simulink model "TorqueVect"  (R2022b)
settings: Solver=ode45  StartTime=0.0  StopTime=inf  RelTol=1e-3  EnableMultiTasking=on
undefined symbols (not defined in the file or in its folder): TC_Decr_Gas, TC_Derivative, TC_Incr_Gas, TC_On, TC_Relay_Off, TC_Relay_On, TV_On, TV_Override
libraries: CarMaker4SL x32, simulink x4, simulink_extras x4
(part 3 of 6)

== system TorqueVect/CarMaker/IPG Vehicle/CarAndTrailer/Forces/Suspension Forces/CreateBus FrcSystemCtrlOutOpt ==
  note: <Your model here>
  In : Inport
  Bus Creator9 : BusCreator  Inputs=64
  Demux : Demux  Outputs=64
  Out : Outport
  wires:
  In/1 -> Demux/1
  Bus Creator9/1 -> Out/1
  Demux/64 -> Bus Creator9/64  "CtrlOutOpt63"
  Demux/1 -> Bus Creator9/1  "CtrlOutOpt0"
  Demux/2 -> Bus Creator9/2  "CtrlOutOpt1"
  Demux/3 -> Bus Creator9/3  "CtrlOutOpt2"
  Demux/4 -> Bus Creator9/4  "CtrlOutOpt3"
  Demux/5 -> Bus Creator9/5  "CtrlOutOpt4"
  Demux/6 -> Bus Creator9/6  "CtrlOutOpt5"
  Demux/7 -> Bus Creator9/7  "CtrlOutOpt6"
  Demux/8 -> Bus Creator9/8  "CtrlOutOpt7"
  Demux/9 -> Bus Creator9/9  "CtrlOutOpt8"
  Demux/10 -> Bus Creator9/10  "CtrlOutOpt9"
  Demux/11 -> Bus Creator9/11  "CtrlOutOpt10"
  Demux/12 -> Bus Creator9/12  "CtrlOutOpt11"
  Demux/13 -> Bus Creator9/13  "CtrlOutOpt12"
  Demux/14 -> Bus Creator9/14  "CtrlOutOpt13"
  Demux/15 -> Bus Creator9/15  "CtrlOutOpt14"
  Demux/16 -> Bus Creator9/16  "CtrlOutOpt15"
  Demux/17 -> Bus Creator9/17  "CtrlOutOpt16"
  Demux/18 -> Bus Creator9/18  "CtrlOutOpt17"
  Demux/19 -> Bus Creator9/19  "CtrlOutOpt18"
  Demux/20 -> Bus Creator9/20  "CtrlOutOpt19"
  Demux/21 -> Bus Creator9/21  "CtrlOutOpt20"
  Demux/22 -> Bus Creator9/22  "CtrlOutOpt21"
  Demux/23 -> Bus Creator9/23  "CtrlOutOpt22"
  Demux/24 -> Bus Creator9/24  "CtrlOutOpt23"
  Demux/25 -> Bus Creator9/25  "CtrlOutOpt24"
  Demux/26 -> Bus Creator9/26  "CtrlOutOpt25"
  Demux/27 -> Bus Creator9/27  "CtrlOutOpt26"
  Demux/28 -> Bus Creator9/28  "CtrlOutOpt27"
  Demux/29 -> Bus Creator9/29  "CtrlOutOpt28"
  Demux/30 -> Bus Creator9/30  "CtrlOutOpt29"
  Demux/31 -> Bus Creator9/31  "CtrlOutOpt30"
  Demux/32 -> Bus Creator9/32  "CtrlOutOpt31"
  Demux/33 -> Bus Creator9/33  "CtrlOutOpt32"
  Demux/34 -> Bus Creator9/34  "CtrlOutOpt33"
  Demux/35 -> Bus Creator9/35  "CtrlOutOpt34"
  Demux/36 -> Bus Creator9/36  "CtrlOutOpt35"
  Demux/37 -> Bus Creator9/37  "CtrlOutOpt36"
  Demux/38 -> Bus Creator9/38  "CtrlOutOpt37"
  Demux/39 -> Bus Creator9/39  "CtrlOutOpt38"
  Demux/40 -> Bus Creator9/40  "CtrlOutOpt39"
  Demux/41 -> Bus Creator9/41  "CtrlOutOpt40"
  Demux/42 -> Bus Creator9/42  "CtrlOutOpt41"
  Demux/43 -> Bus Creator9/43  "CtrlOutOpt42"
  Demux/44 -> Bus Creator9/44  "CtrlOutOpt43"
  Demux/45 -> Bus Creator9/45  "CtrlOutOpt44"
  Demux/46 -> Bus Creator9/46  "CtrlOutOpt45"
  Demux/47 -> Bus Creator9/47  "CtrlOutOpt46"
  Demux/48 -> Bus Creator9/48  "CtrlOutOpt47"
  Demux/49 -> Bus Creator9/49  "CtrlOutOpt48"
  Demux/50 -> Bus Creator9/50  "CtrlOutOpt49"
  Demux/51 -> Bus Creator9/51  "CtrlOutOpt50"
  Demux/52 -> Bus Creator9/52  "CtrlOutOpt51"
  Demux/53 -> Bus Creator9/53  "CtrlOutOpt52"
  Demux/54 -> Bus Creator9/54  "CtrlOutOpt53"
  Demux/55 -> Bus Creator9/55  "CtrlOutOpt54"
  Demux/56 -> Bus Creator9/56  "CtrlOutOpt55"
  Demux/57 -> Bus Creator9/57  "CtrlOutOpt56"
  Demux/58 -> Bus Creator9/58  "CtrlOutOpt57"
  Demux/59 -> Bus Creator9/59  "CtrlOutOpt58"
  Demux/60 -> Bus Creator9/60  "CtrlOutOpt59"
  Demux/61 -> Bus Creator9/61  "CtrlOutOpt60"
  Demux/62 -> Bus Creator9/62  "CtrlOutOpt61"
  Demux/63 -> Bus Creator9/63  "CtrlOutOpt62"

== system TorqueVect/CarMaker/IPG Vehicle/CarAndTrailer/Forces/Suspension Forces/CreateBus SpringCtrlOutOpt ==
  note: <Your model here>
  In : Inport
  Bus Creator{,1..3,9} (5 alike) : BusCreator  Inputs=4
  Demux{,2..5} (5 alike) : Demux
  Out : Outport
  wires:
  Bus Creator/1 -> Bus Creator9/1
  Demux/4 -> Demux5/1  "RR"
  Bus Creator2/1 -> Bus Creator9/3
  Demux5/1 -> Bus Creator3/1  "RR CtrlOutOpt0"
  Bus Creator3/1 -> Bus Creator9/4
  Demux2/4 -> Bus Creator/4  "FL CtrlOutOpt3"
  Demux5/3 -> Bus Creator3/3  "RR CtrlOutOpt2"
  Demux4/3 -> Bus Creator2/3  "RL CtrlOutOpt2"
  Bus Creator1/1 -> Bus Creator9/2
  Demux4/2 -> Bus Creator2/2  "RL CtrlOutOpt1"
  Demux2/2 -> Bus Creator/2  "FL CtrlOutOpt1"
  Demux/2 -> Demux3/1  "FR"
  Demux3/4 -> Bus Creator1/4  "FR CtrlOutOpt3"
  Demux3/1 -> Bus Creator1/1  "FR CtrlOutOpt0"
  Demux4/4 -> Bus Creator2/4  "RL CtrlOutOpt3"
  Demux2/3 -> Bus Creator/3  "FL CtrlOutOpt2"
  Demux3/2 -> Bus Creator1/2  "FR CtrlOutOpt1"
  Demux2/1 -> Bus Creator/1  "FL CtrlOutOpt0"
  Demux3/3 -> Bus Creator1/3  "FR CtrlOutOpt2"
  In/1 -> Demux/1
  Demux5/4 -> Bus Creator3/4  "RR CtrlOutOpt3"
  Demux/3 -> Demux4/1  "RL"
  Bus Creator9/1 -> Out/1
  Demux5/2 -> Bus Creator3/2  "RR CtrlOutOpt1"
  Demux4/1 -> Bus Creator2/1  "RL CtrlOutOpt0"
  Demux/1 -> Demux2/1  "FL"

== system TorqueVect/CarMaker/IPG Vehicle/CarAndTrailer/Forces/Suspension Forces/CreateBus StabiCtrlOutOpt ==
  note: <Your model here>
  In : Inport
  Bus Creator{,1..3,9} (5 alike) : BusCreator  Inputs=4
  Demux{,2..5} (5 alike) : Demux
  Out : Outport
  wires:
  Bus Creator/1 -> Bus Creator9/1
  Demux/4 -> Demux5/1  "RR"
  Bus Creator2/1 -> Bus Creator9/3
  Demux5/1 -> Bus Creator3/1  "RR CtrlOutOpt0"
  Bus Creator3/1 -> Bus Creator9/4
  Demux2/4 -> Bus Creator/4  "FL CtrlOutOpt3"
  Demux5/3 -> Bus Creator3/3  "RR CtrlOutOpt2"
  Demux4/3 -> Bus Creator2/3  "RL CtrlOutOpt2"
  Bus Creator1/1 -> Bus Creator9/2
  Demux4/2 -> Bus Creator2/2  "RL CtrlOutOpt1"
  Demux2/2 -> Bus Creator/2  "FL CtrlOutOpt1"
  Demux/2 -> Demux3/1  "FR"
  Demux3/4 -> Bus Creator1/4  "FR CtrlOutOpt3"
  Demux3/1 -> Bus Creator1/1  "FR CtrlOutOpt0"
  Demux4/4 -> Bus Creator2/4  "RL CtrlOutOpt3"
  Demux2/3 -> Bus Creator/3  "FL CtrlOutOpt2"
  Demux3/2 -> Bus Creator1/2  "FR CtrlOutOpt1"
  Demux2/1 -> Bus Creator/1  "FL CtrlOutOpt0"
  Demux3/3 -> Bus Creator1/3  "FR CtrlOutOpt2"
  In/1 -> Demux/1
  Demux5/4 -> Bus Creator3/4  "RR CtrlOutOpt3"
  Demux/3 -> Demux4/1  "RL"
  Bus Creator9/1 -> Out/1
  Demux5/2 -> Bus Creator3/2  "RR CtrlOutOpt1"
  Demux4/1 -> Bus Creator2/1  "RL CtrlOutOpt0"
  Demux/1 -> Demux2/1  "FL"

== system TorqueVect/CarMaker/IPG Vehicle/CarAndTrailer/Forces/Suspension Forces/CreateBus Suspension Forces ==
  note: <Your model here>
  In : Inport
  Bus Creator10 : BusCreator  Inputs=4
  Bus Creator{4..7} (4 alike) : BusCreator  Inputs=6
  Demux1 : Demux
  Demux{6..9} (4 alike) : Demux  Outputs=6
  Out : Outport
  wires:
  Demux9/5 -> Bus Creator7/5  "RR ParasiticStiffForce"
  Demux9/4 -> Bus Creator7/4  "RR BufferForce"
  Demux6/5 -> Bus Creator4/5  "FL ParasiticStiffForce"
  Demux6/6 -> Bus Creator4/6  "FL ParasiticFricForce"
  Demux1/1 -> Demux6/1  "FL"
  Demux9/1 -> Bus Creator7/1  "RR SpringForce"
  Demux9/6 -> Bus Creator7/6  "RR ParasiticFricForce"
  Demux6/4 -> Bus Creator4/4  "FL BufferForce"
  Demux8/3 -> Bus Creator6/3  "RL StabiForce"
  Demux9/2 -> Bus Creator7/2  "RR DamperForce"
  Demux8/5 -> Bus Creator6/5  "RL ParasiticStiffForce"
  Bus Creator5/1 -> Bus Creator10/2
  Bus Creator6/1 -> Bus Creator10/3
  Bus Creator4/1 -> Bus Creator10/1
  Demux8/4 -> Bus Creator6/4  "RL BufferForce"
  Demux7/1 -> Bus Creator5/1  "FR SpringForce"
  Demux8/6 -> Bus Creator6/6  "RL ParasiticFricForce"
  Demux8/2 -> Bus Creator6/2  "RL DamperForce"
  Demux1/2 -> Demux7/1  "FR"
  Demux6/2 -> Bus Creator4/2  "FL DamperForce"
  Demux1/4 -> Demux9/1  "RR"
  Demux6/1 -> Bus Creator4/1  "FL SpringForce"
  Demux8/1 -> Bus Creator6/1  "RL SpringForce"
  Demux7/3 -> Bus Creator5/3  "FR StabiForce"
  In/1 -> Demux1/1
  Demux7/6 -> Bus Creator5/6  "FR ParasiticFricForce"
  Demux6/3 -> Bus Creator4/3  "FL StabiForce"
  Demux7/2 -> Bus Creator5/2  "FR DamperForce"
  Bus Creator10/1 -> Out/1
  Demux7/5 -> Bus Creator5/5  "FR ParasiticStiffForce"
  Demux7/4 -> Bus Creator5/4  "FR BufferForce"
  Demux9/3 -> Bus Creator7/3  "RR StabiForce"
  Demux1/3 -> Demux8/1  "RL"
  Bus Creator7/1 -> Bus Creator10/4

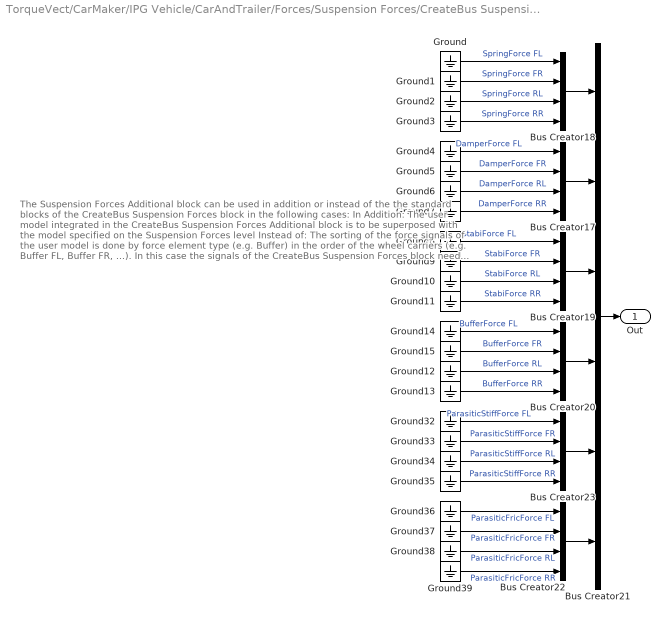
== system TorqueVect/CarMaker/IPG Vehicle/CarAndTrailer/Forces/Suspension Forces/CreateBus Suspension Forces Additional ==
  note: The Suspension Forces Additional block can be used in addition or instead of the
      | the standard blocks of the CreateBus Suspension Forces block in the following cases:
      |
      | In Addition: The user model integrated in the CreateBus Suspension Forces Additional block is to be superposed with the model specified on the Suspension Forces level
      | Instead of: The sorting of the force signals of the user model is done by force element type (e.g. Buffer) in the order of the wheel carriers (e.g. Buffer FL, Buffer FR, ...). In this case the signals of the CreateBus Suspension Forces block need to be disabled e.g. by manually connecting them to ground signals.
      |
      | ATTENTION : The forces given in the CreateBus Suspension Forces Additional block are internally added to the forces of the Suspension Forces block. If this is not desired, make sure to include a force model only in one of the two levels.
  Bus Creator{17..20,22..23} (6 alike) : BusCreator  Inputs=4
  Bus Creator21 : BusCreator  Inputs=6
  Ground{,1..15,32..39} (24 alike) : Ground
  Out : Outport
  wires:
  Ground1/1 -> Bus Creator18/2  "SpringForce FR"
  Ground9/1 -> Bus Creator19/2  "StabiForce FR"
  Ground8/1 -> Bus Creator19/1  "StabiForce FL"
  Bus Creator22/1 -> Bus Creator21/6
  Bus Creator21/1 -> Out/1
  Ground/1 -> Bus Creator18/1  "SpringForce FL"
  Ground36/1 -> Bus Creator22/1  "ParasiticFricForce FL"
  Ground2/1 -> Bus Creator18/3  "SpringForce RL"
  Ground5/1 -> Bus Creator17/2  "DamperForce FR"
  Ground15/1 -> Bus Creator20/2  "BufferForce FR"
  Ground35/1 -> Bus Creator23/4  "ParasiticStiffForce RR"
  Bus Creator20/1 -> Bus Creator21/4
  Bus Creator17/1 -> Bus Creator21/2
  Ground37/1 -> Bus Creator22/2  "ParasiticFricForce FR"
  Ground4/1 -> Bus Creator17/1  "DamperForce FL"
  Ground33/1 -> Bus Creator23/2  "ParasiticStiffForce FR"
  Bus Creator23/1 -> Bus Creator21/5
  Ground11/1 -> Bus Creator19/4  "StabiForce RR"
  Ground10/1 -> Bus Creator19/3  "StabiForce RL"
  Ground6/1 -> Bus Creator17/3  "DamperForce RL"
  Bus Creator19/1 -> Bus Creator21/3
  Ground7/1 -> Bus Creator17/4  "DamperForce RR"
  Bus Creator18/1 -> Bus Creator21/1
  Ground34/1 -> Bus Creator23/3  "ParasiticStiffForce RL"
  Ground3/1 -> Bus Creator18/4  "SpringForce RR"
  Ground12/1 -> Bus Creator20/3  "BufferForce RL"
  Ground38/1 -> Bus Creator22/3  "ParasiticFricForce RL"
  Ground14/1 -> Bus Creator20/1  "BufferForce FL"
  Ground39/1 -> Bus Creator22/4  "ParasiticFricForce RR"
  Ground32/1 -> Bus Creator23/1  "ParasiticStiffForce FL"
  Ground13/1 -> Bus Creator20/4  "BufferForce RR"

== system TorqueVect/CarMaker/IPG Vehicle/CarAndTrailer/Forces/Suspension Forces/CreateBus Suspension Forces CtrlOut ==
  note: <Your model here>
  In : Inport
  Bus Creator{,1..3,9} (5 alike) : BusCreator  Inputs=4
  Demux{,2..5} (5 alike) : Demux
  Out : Outport
  wires:
  Bus Creator3/1 -> Bus Creator9/4
  Demux2/4 -> Bus Creator/4  "FL BufferCtrlOut"
  Demux/4 -> Demux5/1  "RR"
  Bus Creator2/1 -> Bus Creator9/3
  Demux3/1 -> Bus Creator1/1  "FR SpringCtrlOut"
  Bus Creator/1 -> Bus Creator9/1
  Demux5/1 -> Bus Creator3/1  "RR SpringCtrlOut"
  Demux5/2 -> Bus Creator3/2  "RR DamperCtrlOut"
  Demux4/2 -> Bus Creator2/2  "RL DamperCtrlOut"
  Demux4/3 -> Bus Creator2/3  "RL StabiCtrlOut"
  Demux2/2 -> Bus Creator/2  "FL DamperCtrlOut"
  Demux/3 -> Demux4/1  "RL"
  Demux5/4 -> Bus Creator3/4  "RR BufferCtrlOut"
  In/1 -> Demux/1
  Demux2/1 -> Bus Creator/1  "FL SpringCtrlOut"
  Demux3/3 -> Bus Creator1/3  "FR StabiCtrlOut"
  Demux3/2 -> Bus Creator1/2  "FR DamperCtrlOut"
  Demux4/1 -> Bus Creator2/1  "RL SpringCtrlOut"
  Demux4/4 -> Bus Creator2/4  "RL BufferCtrlOut"
  Demux2/3 -> Bus Creator/3  "FL StabiCtrlOut"
  Bus Creator1/1 -> Bus Creator9/2
  Bus Creator9/1 -> Out/1
  Demux/1 -> Demux2/1  "FL"
  Demux/2 -> Demux3/1  "FR"
  Demux5/3 -> Bus Creator3/3  "RR StabiCtrlOut"
  Demux3/4 -> Bus Creator1/4  "FR BufferCtrlOut"

== system TorqueVect/CarMaker/IPG Vehicle/CarAndTrailer/Forces/Suspension Forces/Damper CreateBus CtrlOutOpt ==
  note: <Your model here>
  In : Inport
  Bus Creator{,1..3,9} (5 alike) : BusCreator  Inputs=4
  Demux{,2..5} (5 alike) : Demux
  Out : Outport
  wires:
  Bus Creator/1 -> Bus Creator9/1
  Demux/4 -> Demux5/1  "RR"
  Bus Creator2/1 -> Bus Creator9/3
  Demux5/1 -> Bus Creator3/1  "RR CtrlOutOpt0"
  Bus Creator3/1 -> Bus Creator9/4
  Demux2/4 -> Bus Creator/4  "FL CtrlOutOpt3"
  Demux5/3 -> Bus Creator3/3  "RR CtrlOutOpt2"
  Demux4/3 -> Bus Creator2/3  "RL CtrlOutOpt2"
  Bus Creator1/1 -> Bus Creator9/2
  Demux4/2 -> Bus Creator2/2  "RL CtrlOutOpt1"
  Demux2/2 -> Bus Creator/2  "FL CtrlOutOpt1"
  Demux/2 -> Demux3/1  "FR"
  Demux3/4 -> Bus Creator1/4  "FR CtrlOutOpt3"
  Demux3/1 -> Bus Creator1/1  "FR CtrlOutOpt0"
  Demux4/4 -> Bus Creator2/4  "RL CtrlOutOpt3"
  Demux2/3 -> Bus Creator/3  "FL CtrlOutOpt2"
  Demux3/2 -> Bus Creator1/2  "FR CtrlOutOpt1"
  Demux2/1 -> Bus Creator/1  "FL CtrlOutOpt0"
  Demux3/3 -> Bus Creator1/3  "FR CtrlOutOpt2"
  In/1 -> Demux/1
  Demux5/4 -> Bus Creator3/4  "RR CtrlOutOpt3"
  Demux/3 -> Demux4/1  "RL"
  Bus Creator9/1 -> Out/1
  Demux5/2 -> Bus Creator3/2  "RR CtrlOutOpt1"
  Demux4/1 -> Bus Creator2/1  "RL CtrlOutOpt0"
  Demux/1 -> Demux2/1  "FL"

== system TorqueVect/CarMaker/IPG Vehicle/CarAndTrailer/Forces/Suspension Forces/FrcSystem CreateBus CtrlOutOpt ==
  note: <Your model here>
  In : Inport
  Bus Creator9 : BusCreator  Inputs=64
  Demux : Demux  Outputs=64
  Out : Outport
  wires:
  In/1 -> Demux/1
  Bus Creator9/1 -> Out/1
  Demux/64 -> Bus Creator9/64  "CtrlOutOpt63"
  Demux/1 -> Bus Creator9/1  "CtrlOutOpt0"
  Demux/2 -> Bus Creator9/2  "CtrlOutOpt1"
  Demux/3 -> Bus Creator9/3  "CtrlOutOpt2"
  Demux/4 -> Bus Creator9/4  "CtrlOutOpt3"
  Demux/5 -> Bus Creator9/5  "CtrlOutOpt4"
  Demux/6 -> Bus Creator9/6  "CtrlOutOpt5"
  Demux/7 -> Bus Creator9/7  "CtrlOutOpt6"
  Demux/8 -> Bus Creator9/8  "CtrlOutOpt7"
  Demux/9 -> Bus Creator9/9  "CtrlOutOpt8"
  Demux/10 -> Bus Creator9/10  "CtrlOutOpt9"
  Demux/11 -> Bus Creator9/11  "CtrlOutOpt10"
  Demux/12 -> Bus Creator9/12  "CtrlOutOpt11"
  Demux/13 -> Bus Creator9/13  "CtrlOutOpt12"
  Demux/14 -> Bus Creator9/14  "CtrlOutOpt13"
  Demux/15 -> Bus Creator9/15  "CtrlOutOpt14"
  Demux/16 -> Bus Creator9/16  "CtrlOutOpt15"
  Demux/17 -> Bus Creator9/17  "CtrlOutOpt16"
  Demux/18 -> Bus Creator9/18  "CtrlOutOpt17"
  Demux/19 -> Bus Creator9/19  "CtrlOutOpt18"
  Demux/20 -> Bus Creator9/20  "CtrlOutOpt19"
  Demux/21 -> Bus Creator9/21  "CtrlOutOpt20"
  Demux/22 -> Bus Creator9/22  "CtrlOutOpt21"
  Demux/23 -> Bus Creator9/23  "CtrlOutOpt22"
  Demux/24 -> Bus Creator9/24  "CtrlOutOpt23"
  Demux/25 -> Bus Creator9/25  "CtrlOutOpt24"
  Demux/26 -> Bus Creator9/26  "CtrlOutOpt25"
  Demux/27 -> Bus Creator9/27  "CtrlOutOpt26"
  Demux/28 -> Bus Creator9/28  "CtrlOutOpt27"
  Demux/29 -> Bus Creator9/29  "CtrlOutOpt28"
  Demux/30 -> Bus Creator9/30  "CtrlOutOpt29"
  Demux/31 -> Bus Creator9/31  "CtrlOutOpt30"
  Demux/32 -> Bus Creator9/32  "CtrlOutOpt31"
  Demux/33 -> Bus Creator9/33  "CtrlOutOpt32"
  Demux/34 -> Bus Creator9/34  "CtrlOutOpt33"
  Demux/35 -> Bus Creator9/35  "CtrlOutOpt34"
  Demux/36 -> Bus Creator9/36  "CtrlOutOpt35"
  Demux/37 -> Bus Creator9/37  "CtrlOutOpt36"
  Demux/38 -> Bus Creator9/38  "CtrlOutOpt37"
  Demux/39 -> Bus Creator9/39  "CtrlOutOpt38"
  Demux/40 -> Bus Creator9/40  "CtrlOutOpt39"
  Demux/41 -> Bus Creator9/41  "CtrlOutOpt40"
  Demux/42 -> Bus Creator9/42  "CtrlOutOpt41"
  Demux/43 -> Bus Creator9/43  "CtrlOutOpt42"
  Demux/44 -> Bus Creator9/44  "CtrlOutOpt43"
  Demux/45 -> Bus Creator9/45  "CtrlOutOpt44"
  Demux/46 -> Bus Creator9/46  "CtrlOutOpt45"
  Demux/47 -> Bus Creator9/47  "CtrlOutOpt46"
  Demux/48 -> Bus Creator9/48  "CtrlOutOpt47"
  Demux/49 -> Bus Creator9/49  "CtrlOutOpt48"
  Demux/50 -> Bus Creator9/50  "CtrlOutOpt49"
  Demux/51 -> Bus Creator9/51  "CtrlOutOpt50"
  Demux/52 -> Bus Creator9/52  "CtrlOutOpt51"
  Demux/53 -> Bus Creator9/53  "CtrlOutOpt52"
  Demux/54 -> Bus Creator9/54  "CtrlOutOpt53"
  Demux/55 -> Bus Creator9/55  "CtrlOutOpt54"
  Demux/56 -> Bus Creator9/56  "CtrlOutOpt55"
  Demux/57 -> Bus Creator9/57  "CtrlOutOpt56"
  Demux/58 -> Bus Creator9/58  "CtrlOutOpt57"
  Demux/59 -> Bus Creator9/59  "CtrlOutOpt58"
  Demux/60 -> Bus Creator9/60  "CtrlOutOpt59"
  Demux/61 -> Bus Creator9/61  "CtrlOutOpt60"
  Demux/62 -> Bus Creator9/62  "CtrlOutOpt61"
  Demux/63 -> Bus Creator9/63  "CtrlOutOpt62"

== system TorqueVect/CarMaker/IPG Vehicle/CarAndTrailer/Forces/Suspension Forces/Spring CreateBus CtrlOutOpt ==
  note: <Your model here>
  In : Inport
  Bus Creator{,1..3,9} (5 alike) : BusCreator  Inputs=4
  Demux{,2..5} (5 alike) : Demux
  Out : Outport
  wires:
  Bus Creator/1 -> Bus Creator9/1
  Demux/4 -> Demux5/1  "RR"
  Bus Creator2/1 -> Bus Creator9/3
  Demux5/1 -> Bus Creator3/1  "RR CtrlOutOpt0"
  Bus Creator3/1 -> Bus Creator9/4
  Demux2/4 -> Bus Creator/4  "FL CtrlOutOpt3"
  Demux5/3 -> Bus Creator3/3  "RR CtrlOutOpt2"
  Demux4/3 -> Bus Creator2/3  "RL CtrlOutOpt2"
  Bus Creator1/1 -> Bus Creator9/2
  Demux4/2 -> Bus Creator2/2  "RL CtrlOutOpt1"
  Demux2/2 -> Bus Creator/2  "FL CtrlOutOpt1"
  Demux/2 -> Demux3/1  "FR"
  Demux3/4 -> Bus Creator1/4  "FR CtrlOutOpt3"
  Demux3/1 -> Bus Creator1/1  "FR CtrlOutOpt0"
  Demux4/4 -> Bus Creator2/4  "RL CtrlOutOpt3"
  Demux2/3 -> Bus Creator/3  "FL CtrlOutOpt2"
  Demux3/2 -> Bus Creator1/2  "FR CtrlOutOpt1"
  Demux2/1 -> Bus Creator/1  "FL CtrlOutOpt0"
  Demux3/3 -> Bus Creator1/3  "FR CtrlOutOpt2"
  In/1 -> Demux/1
  Demux5/4 -> Bus Creator3/4  "RR CtrlOutOpt3"
  Demux/3 -> Demux4/1  "RL"
  Bus Creator9/1 -> Out/1
  Demux5/2 -> Bus Creator3/2  "RR CtrlOutOpt1"
  Demux4/1 -> Bus Creator2/1  "RL CtrlOutOpt0"
  Demux/1 -> Demux2/1  "FL"

== system TorqueVect/CarMaker/IPG Vehicle/CarAndTrailer/Forces/Suspension Forces/Stabi CreateBus CtrlOutOpt ==
  note: <Your model here>
  In : Inport
  Bus Creator{,1..3,9} (5 alike) : BusCreator  Inputs=4
  Demux{,2..5} (5 alike) : Demux
  Out : Outport
  wires:
  Bus Creator/1 -> Bus Creator9/1
  Demux/4 -> Demux5/1  "RR"
  Bus Creator2/1 -> Bus Creator9/3
  Demux5/1 -> Bus Creator3/1  "RR CtrlOutOpt0"
  Bus Creator3/1 -> Bus Creator9/4
  Demux2/4 -> Bus Creator/4  "FL CtrlOutOpt3"
  Demux5/3 -> Bus Creator3/3  "RR CtrlOutOpt2"
  Demux4/3 -> Bus Creator2/3  "RL CtrlOutOpt2"
  Bus Creator1/1 -> Bus Creator9/2
  Demux4/2 -> Bus Creator2/2  "RL CtrlOutOpt1"
  Demux2/2 -> Bus Creator/2  "FL CtrlOutOpt1"
  Demux/2 -> Demux3/1  "FR"
  Demux3/4 -> Bus Creator1/4  "FR CtrlOutOpt3"
  Demux3/1 -> Bus Creator1/1  "FR CtrlOutOpt0"
  Demux4/4 -> Bus Creator2/4  "RL CtrlOutOpt3"
  Demux2/3 -> Bus Creator/3  "FL CtrlOutOpt2"
  Demux3/2 -> Bus Creator1/2  "FR CtrlOutOpt1"
  Demux2/1 -> Bus Creator/1  "FL CtrlOutOpt0"
  Demux3/3 -> Bus Creator1/3  "FR CtrlOutOpt2"
  In/1 -> Demux/1
  Demux5/4 -> Bus Creator3/4  "RR CtrlOutOpt3"
  Demux/3 -> Demux4/1  "RL"
  Bus Creator9/1 -> Out/1
  Demux5/2 -> Bus Creator3/2  "RR CtrlOutOpt1"
  Demux4/1 -> Bus Creator2/1  "RL CtrlOutOpt0"
  Demux/1 -> Demux2/1  "FL"

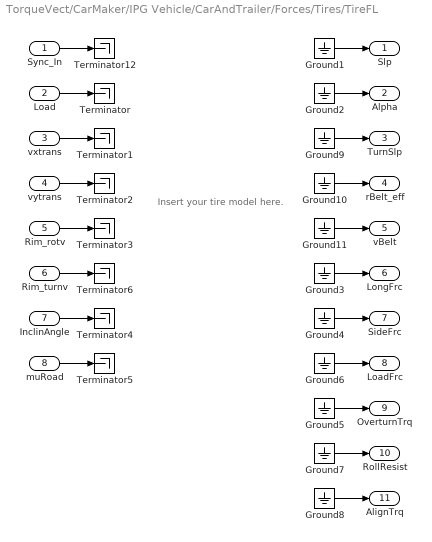
== system TorqueVect/CarMaker/IPG Vehicle/CarAndTrailer/Forces/Tires/TireFL ==
  note: Insert your tire model here.
  Sync_In : Inport
  Load : Inport  Port=2
  vxtrans : Inport  Port=3
  vytrans : Inport  Port=4
  Rim_rotv : Inport  Port=5
  Rim_turnv : Inport  Port=6
  InclinAngle : Inport  Port=7
  muRoad : Inport  Port=8
  Ground{1..11} (11 alike) : Ground
  Terminator{,1..6,12} (8 alike) : Terminator
  Slp : Outport  VectorParamsAs1DForOutWhenUnconnected=off
  Alpha : Outport  Port=2  VectorParamsAs1DForOutWhenUnconnected=off
  TurnSlp : Outport  Port=3  VectorParamsAs1DForOutWhenUnconnected=off
  rBelt_eff : Outport  Port=4  VectorParamsAs1DForOutWhenUnconnected=off
  vBelt : Outport  Port=5  VectorParamsAs1DForOutWhenUnconnected=off
  LongFrc : Outport  Port=6  VectorParamsAs1DForOutWhenUnconnected=off
  SideFrc : Outport  Port=7  VectorParamsAs1DForOutWhenUnconnected=off
  LoadFrc : Outport  Port=8  VectorParamsAs1DForOutWhenUnconnected=off
  OverturnTrq : Outport  Port=9  VectorParamsAs1DForOutWhenUnconnected=off
  RollResist : Outport  Port=10  VectorParamsAs1DForOutWhenUnconnected=off
  AlignTrq : Outport  Port=11  VectorParamsAs1DForOutWhenUnconnected=off
  wires:
  Ground11/1 -> vBelt/1
  Ground10/1 -> rBelt_eff/1
  Ground9/1 -> TurnSlp/1
  Rim_turnv/1 -> Terminator6/1
  Sync_In/1 -> Terminator12/1
  Ground2/1 -> Alpha/1
  Ground3/1 -> LongFrc/1
  Ground4/1 -> SideFrc/1
  Ground5/1 -> OverturnTrq/1
  vxtrans/1 -> Terminator1/1
  vytrans/1 -> Terminator2/1
  Rim_rotv/1 -> Terminator3/1
  InclinAngle/1 -> Terminator4/1
  muRoad/1 -> Terminator5/1
  Load/1 -> Terminator/1
  Ground1/1 -> Slp/1
  Ground6/1 -> LoadFrc/1
  Ground7/1 -> RollResist/1
  Ground8/1 -> AlignTrq/1

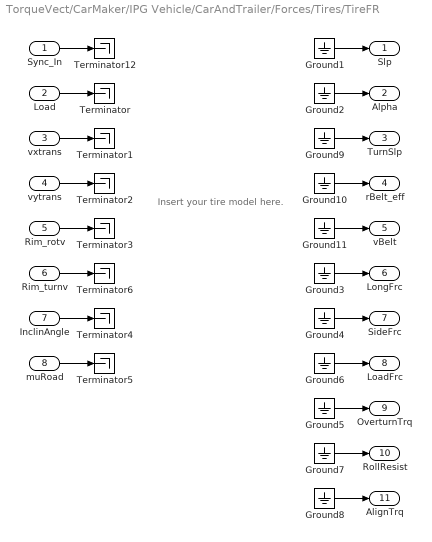
== system TorqueVect/CarMaker/IPG Vehicle/CarAndTrailer/Forces/Tires/TireFR ==
  note: Insert your tire model here.
  Sync_In : Inport
  Load : Inport  Port=2
  vxtrans : Inport  Port=3
  vytrans : Inport  Port=4
  Rim_rotv : Inport  Port=5
  Rim_turnv : Inport  Port=6
  InclinAngle : Inport  Port=7
  muRoad : Inport  Port=8
  Ground{1..11} (11 alike) : Ground
  Terminator{,1..6,12} (8 alike) : Terminator
  Slp : Outport  VectorParamsAs1DForOutWhenUnconnected=off
  Alpha : Outport  Port=2  VectorParamsAs1DForOutWhenUnconnected=off
  TurnSlp : Outport  Port=3  VectorParamsAs1DForOutWhenUnconnected=off
  rBelt_eff : Outport  Port=4  VectorParamsAs1DForOutWhenUnconnected=off
  vBelt : Outport  Port=5  VectorParamsAs1DForOutWhenUnconnected=off
  LongFrc : Outport  Port=6  VectorParamsAs1DForOutWhenUnconnected=off
  SideFrc : Outport  Port=7  VectorParamsAs1DForOutWhenUnconnected=off
  LoadFrc : Outport  Port=8  VectorParamsAs1DForOutWhenUnconnected=off
  OverturnTrq : Outport  Port=9  VectorParamsAs1DForOutWhenUnconnected=off
  RollResist : Outport  Port=10  VectorParamsAs1DForOutWhenUnconnected=off
  AlignTrq : Outport  Port=11  VectorParamsAs1DForOutWhenUnconnected=off
  wires:
  Ground11/1 -> vBelt/1
  Ground10/1 -> rBelt_eff/1
  Ground9/1 -> TurnSlp/1
  Rim_turnv/1 -> Terminator6/1
  Sync_In/1 -> Terminator12/1
  Ground2/1 -> Alpha/1
  Ground3/1 -> LongFrc/1
  Ground4/1 -> SideFrc/1
  Ground5/1 -> OverturnTrq/1
  vxtrans/1 -> Terminator1/1
  vytrans/1 -> Terminator2/1
  Rim_rotv/1 -> Terminator3/1
  InclinAngle/1 -> Terminator4/1
  muRoad/1 -> Terminator5/1
  Load/1 -> Terminator/1
  Ground1/1 -> Slp/1
  Ground6/1 -> LoadFrc/1
  Ground7/1 -> RollResist/1
  Ground8/1 -> AlignTrq/1

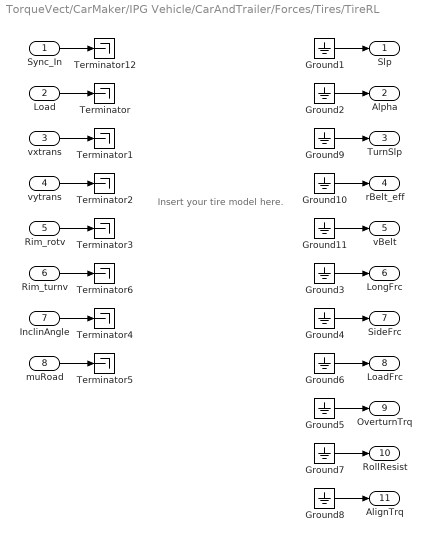
== system TorqueVect/CarMaker/IPG Vehicle/CarAndTrailer/Forces/Tires/TireRL ==
  note: Insert your tire model here.
  Sync_In : Inport
  Load : Inport  Port=2
  vxtrans : Inport  Port=3
  vytrans : Inport  Port=4
  Rim_rotv : Inport  Port=5
  Rim_turnv : Inport  Port=6
  InclinAngle : Inport  Port=7
  muRoad : Inport  Port=8
  Ground{1..11} (11 alike) : Ground
  Terminator{,1..6,12} (8 alike) : Terminator
  Slp : Outport  VectorParamsAs1DForOutWhenUnconnected=off
  Alpha : Outport  Port=2  VectorParamsAs1DForOutWhenUnconnected=off
  TurnSlp : Outport  Port=3  VectorParamsAs1DForOutWhenUnconnected=off
  rBelt_eff : Outport  Port=4  VectorParamsAs1DForOutWhenUnconnected=off
  vBelt : Outport  Port=5  VectorParamsAs1DForOutWhenUnconnected=off
  LongFrc : Outport  Port=6  VectorParamsAs1DForOutWhenUnconnected=off
  SideFrc : Outport  Port=7  VectorParamsAs1DForOutWhenUnconnected=off
  LoadFrc : Outport  Port=8  VectorParamsAs1DForOutWhenUnconnected=off
  OverturnTrq : Outport  Port=9  VectorParamsAs1DForOutWhenUnconnected=off
  RollResist : Outport  Port=10  VectorParamsAs1DForOutWhenUnconnected=off
  AlignTrq : Outport  Port=11  VectorParamsAs1DForOutWhenUnconnected=off
  wires:
  Ground11/1 -> vBelt/1
  Ground10/1 -> rBelt_eff/1
  Ground9/1 -> TurnSlp/1
  Rim_turnv/1 -> Terminator6/1
  Sync_In/1 -> Terminator12/1
  Ground2/1 -> Alpha/1
  Ground3/1 -> LongFrc/1
  Ground4/1 -> SideFrc/1
  Ground5/1 -> OverturnTrq/1
  vxtrans/1 -> Terminator1/1
  vytrans/1 -> Terminator2/1
  Rim_rotv/1 -> Terminator3/1
  InclinAngle/1 -> Terminator4/1
  muRoad/1 -> Terminator5/1
  Load/1 -> Terminator/1
  Ground1/1 -> Slp/1
  Ground6/1 -> LoadFrc/1
  Ground7/1 -> RollResist/1
  Ground8/1 -> AlignTrq/1

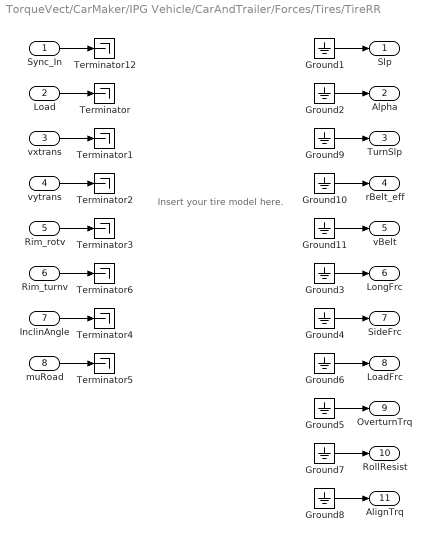
== system TorqueVect/CarMaker/IPG Vehicle/CarAndTrailer/Forces/Tires/TireRR ==
  note: Insert your tire model here.
  Sync_In : Inport
  Load : Inport  Port=2
  vxtrans : Inport  Port=3
  vytrans : Inport  Port=4
  Rim_rotv : Inport  Port=5
  Rim_turnv : Inport  Port=6
  InclinAngle : Inport  Port=7
  muRoad : Inport  Port=8
  Ground{1..11} (11 alike) : Ground
  Terminator{,1..6,12} (8 alike) : Terminator
  Slp : Outport  VectorParamsAs1DForOutWhenUnconnected=off
  Alpha : Outport  Port=2  VectorParamsAs1DForOutWhenUnconnected=off
  TurnSlp : Outport  Port=3  VectorParamsAs1DForOutWhenUnconnected=off
  rBelt_eff : Outport  Port=4  VectorParamsAs1DForOutWhenUnconnected=off
  vBelt : Outport  Port=5  VectorParamsAs1DForOutWhenUnconnected=off
  LongFrc : Outport  Port=6  VectorParamsAs1DForOutWhenUnconnected=off
  SideFrc : Outport  Port=7  VectorParamsAs1DForOutWhenUnconnected=off
  LoadFrc : Outport  Port=8  VectorParamsAs1DForOutWhenUnconnected=off
  OverturnTrq : Outport  Port=9  VectorParamsAs1DForOutWhenUnconnected=off
  RollResist : Outport  Port=10  VectorParamsAs1DForOutWhenUnconnected=off
  AlignTrq : Outport  Port=11  VectorParamsAs1DForOutWhenUnconnected=off
  wires:
  Ground11/1 -> vBelt/1
  Ground10/1 -> rBelt_eff/1
  Ground9/1 -> TurnSlp/1
  Rim_turnv/1 -> Terminator6/1
  Sync_In/1 -> Terminator12/1
  Ground2/1 -> Alpha/1
  Ground3/1 -> LongFrc/1
  Ground4/1 -> SideFrc/1
  Ground5/1 -> OverturnTrq/1
  vxtrans/1 -> Terminator1/1
  vytrans/1 -> Terminator2/1
  Rim_rotv/1 -> Terminator3/1
  InclinAngle/1 -> Terminator4/1
  muRoad/1 -> Terminator5/1
  Load/1 -> Terminator/1
  Ground1/1 -> Slp/1
  Ground6/1 -> LoadFrc/1
  Ground7/1 -> RollResist/1
  Ground8/1 -> AlignTrq/1

== system TorqueVect/CarMaker/IPG Vehicle/PowerTrain/PTControl Example/PTC ClutchOut/CreateBus PTC ClutchOut0 ==
  In : Inport
  BusCreator : BusCreator  Inputs=3
  Demux : Demux  Outputs=3
      settings: DisplayOption=none
  Out : Outport  VectorParamsAs1DForOutWhenUnconnected=off
  wires:
  Demux/3 -> BusCreator/3  "PTC ClutchOut0 Trq_out_trg"
  Demux/2 -> BusCreator/2  "PTC ClutchOut0 rotv_out_trg"
  Demux/1 -> BusCreator/1  "PTC ClutchOut0 Pos"
  BusCreator/1 -> Out/1
  In/1 -> Demux/1

== system TorqueVect/CarMaker/IPG Vehicle/PowerTrain/PTControl Example/PTC ClutchOut/CreateBus PTC ClutchOut1 ==
  In : Inport
  BusCreator : BusCreator  Inputs=3
  Demux : Demux  Outputs=3
      settings: DisplayOption=none
  Out : Outport  VectorParamsAs1DForOutWhenUnconnected=off
  wires:
  Demux/3 -> BusCreator/3  "PTC ClutchOut1 Trq_out_trg"
  Demux/2 -> BusCreator/2  "PTC ClutchOut1 rotv_out_trg"
  Demux/1 -> BusCreator/1  "PTC ClutchOut1 Pos"
  BusCreator/1 -> Out/1
  In/1 -> Demux/1

== system TorqueVect/CarMaker/IPG Vehicle/PowerTrain/PTControl Example/PTC ClutchOut/CreateBus PTC ClutchOut10 ==
  In : Inport
  BusCreator : BusCreator  Inputs=3
  Demux : Demux  Outputs=3
      settings: DisplayOption=none
  Out : Outport  VectorParamsAs1DForOutWhenUnconnected=off
  wires:
  Demux/3 -> BusCreator/3  "PTC ClutchOut10 Trq_out_trg"
  Demux/2 -> BusCreator/2  "PTC ClutchOut10 rotv_out_trg"
  Demux/1 -> BusCreator/1  "PTC ClutchOut10 Pos"
  BusCreator/1 -> Out/1
  In/1 -> Demux/1

== system TorqueVect/CarMaker/IPG Vehicle/PowerTrain/PTControl Example/PTC ClutchOut/CreateBus PTC ClutchOut11 ==
  In : Inport
  BusCreator : BusCreator  Inputs=3
  Demux : Demux  Outputs=3
      settings: DisplayOption=none
  Out : Outport  VectorParamsAs1DForOutWhenUnconnected=off
  wires:
  Demux/3 -> BusCreator/3  "PTC ClutchOut11 Trq_out_trg"
  Demux/2 -> BusCreator/2  "PTC ClutchOut11 rotv_out_trg"
  Demux/1 -> BusCreator/1  "PTC ClutchOut11 Pos"
  BusCreator/1 -> Out/1
  In/1 -> Demux/1

== system TorqueVect/CarMaker/IPG Vehicle/PowerTrain/PTControl Example/PTC ClutchOut/CreateBus PTC ClutchOut2 ==
  In : Inport
  BusCreator : BusCreator  Inputs=3
  Demux : Demux  Outputs=3
      settings: DisplayOption=none
  Out : Outport  VectorParamsAs1DForOutWhenUnconnected=off
  wires:
  Demux/3 -> BusCreator/3  "PTC ClutchOut2 Trq_out_trg"
  Demux/2 -> BusCreator/2  "PTC ClutchOut2 rotv_out_trg"
  Demux/1 -> BusCreator/1  "PTC ClutchOut2 Pos"
  BusCreator/1 -> Out/1
  In/1 -> Demux/1

== system TorqueVect/CarMaker/IPG Vehicle/PowerTrain/PTControl Example/PTC ClutchOut/CreateBus PTC ClutchOut3 ==
  In : Inport
  BusCreator : BusCreator  Inputs=3
  Demux : Demux  Outputs=3
      settings: DisplayOption=none
  Out : Outport  VectorParamsAs1DForOutWhenUnconnected=off
  wires:
  Demux/3 -> BusCreator/3  "PTC ClutchOut3 Trq_out_trg"
  Demux/2 -> BusCreator/2  "PTC ClutchOut3 rotv_out_trg"
  Demux/1 -> BusCreator/1  "PTC ClutchOut3 Pos"
  BusCreator/1 -> Out/1
  In/1 -> Demux/1

== system TorqueVect/CarMaker/IPG Vehicle/PowerTrain/PTControl Example/PTC ClutchOut/CreateBus PTC ClutchOut4 ==
  In : Inport
  BusCreator : BusCreator  Inputs=3
  Demux : Demux  Outputs=3
      settings: DisplayOption=none
  Out : Outport  VectorParamsAs1DForOutWhenUnconnected=off
  wires:
  Demux/3 -> BusCreator/3  "PTC ClutchOut4 Trq_out_trg"
  Demux/2 -> BusCreator/2  "PTC ClutchOut4 rotv_out_trg"
  Demux/1 -> BusCreator/1  "PTC ClutchOut4 Pos"
  BusCreator/1 -> Out/1
  In/1 -> Demux/1

== system TorqueVect/CarMaker/IPG Vehicle/PowerTrain/PTControl Example/PTC ClutchOut/CreateBus PTC ClutchOut5 ==
  In : Inport
  BusCreator : BusCreator  Inputs=3
  Demux : Demux  Outputs=3
      settings: DisplayOption=none
  Out : Outport  VectorParamsAs1DForOutWhenUnconnected=off
  wires:
  Demux/3 -> BusCreator/3  "PTC ClutchOut5 Trq_out_trg"
  Demux/2 -> BusCreator/2  "PTC ClutchOut5 rotv_out_trg"
  Demux/1 -> BusCreator/1  "PTC ClutchOut5 Pos"
  BusCreator/1 -> Out/1
  In/1 -> Demux/1

== system TorqueVect/CarMaker/IPG Vehicle/PowerTrain/PTControl Example/PTC ClutchOut/CreateBus PTC ClutchOut6 ==
  In : Inport
  BusCreator : BusCreator  Inputs=3
  Demux : Demux  Outputs=3
      settings: DisplayOption=none
  Out : Outport  VectorParamsAs1DForOutWhenUnconnected=off
  wires:
  Demux/3 -> BusCreator/3  "PTC ClutchOut6 Trq_out_trg"
  Demux/2 -> BusCreator/2  "PTC ClutchOut6 rotv_out_trg"
  Demux/1 -> BusCreator/1  "PTC ClutchOut6 Pos"
  BusCreator/1 -> Out/1
  In/1 -> Demux/1

== system TorqueVect/CarMaker/IPG Vehicle/PowerTrain/PTControl Example/PTC ClutchOut/CreateBus PTC ClutchOut7 ==
  In : Inport
  BusCreator : BusCreator  Inputs=3
  Demux : Demux  Outputs=3
      settings: DisplayOption=none
  Out : Outport  VectorParamsAs1DForOutWhenUnconnected=off
  wires:
  Demux/3 -> BusCreator/3  "PTC ClutchOut7 Trq_out_trg"
  Demux/2 -> BusCreator/2  "PTC ClutchOut7 rotv_out_trg"
  Demux/1 -> BusCreator/1  "PTC ClutchOut7 Pos"
  BusCreator/1 -> Out/1
  In/1 -> Demux/1

== system TorqueVect/CarMaker/IPG Vehicle/PowerTrain/PTControl Example/PTC ClutchOut/CreateBus PTC ClutchOut8 ==
  In : Inport
  BusCreator : BusCreator  Inputs=3
  Demux : Demux  Outputs=3
      settings: DisplayOption=none
  Out : Outport  VectorParamsAs1DForOutWhenUnconnected=off
  wires:
  Demux/3 -> BusCreator/3  "PTC ClutchOut8 Trq_out_trg"
  Demux/2 -> BusCreator/2  "PTC ClutchOut8 rotv_out_trg"
  Demux/1 -> BusCreator/1  "PTC ClutchOut8 Pos"
  BusCreator/1 -> Out/1
  In/1 -> Demux/1

== system TorqueVect/CarMaker/IPG Vehicle/PowerTrain/PTControl Example/PTC ClutchOut/CreateBus PTC ClutchOut9 ==
  In : Inport
  BusCreator : BusCreator  Inputs=3
  Demux : Demux  Outputs=3
      settings: DisplayOption=none
  Out : Outport  VectorParamsAs1DForOutWhenUnconnected=off
  wires:
  Demux/3 -> BusCreator/3  "PTC ClutchOut9 Trq_out_trg"
  Demux/2 -> BusCreator/2  "PTC ClutchOut9 rotv_out_trg"
  Demux/1 -> BusCreator/1  "PTC ClutchOut9 Pos"
  BusCreator/1 -> Out/1
  In/1 -> Demux/1

== system TorqueVect/CarMaker/IPG Vehicle/PowerTrain/PTControl Example/PTC GearBoxOut/CreateBus PTC GearboxOut0 ==
  In : Inport
  BusCreator : BusCreator  Inputs=12
  Demux : Demux  Outputs=12
      settings: DisplayOption=none
  Out : Outport  VectorParamsAs1DForOutWhenUnconnected=off
  wires:
  Demux/12 -> BusCreator/12  "PTC GearboxOut0 Clutch_dis Trq_out_trg"
  Demux/11 -> BusCreator/11  "PTC GearboxOut0 Clutch_dis rotv_out_trg"
  Demux/10 -> BusCreator/10  "PTC GearboxOut0 Clutch_dis Pos"
  Demux/9 -> BusCreator/9  "PTC GearboxOut0 Clutch Trq_out_trg"
  Demux/8 -> BusCreator/8  "PTC GearboxOut0 Clutch rotv_out_trg"
  Demux/7 -> BusCreator/7  "PTC GearboxOut0 Clutch Pos"
  Demux/6 -> BusCreator/6  "PTC GearboxOut0 Trq_out_trg"
  Demux/5 -> BusCreator/5  "PTC GearboxOut0 rotv_in_trg"
  Demux/4 -> BusCreator/4  "PTC GearboxOut0 i_trg"
  Demux/3 -> BusCreator/3  "PTC GearboxOut0 set_ParkBrake"
  Demux/2 -> BusCreator/2  "PTC GearboxOut0 GearNoTrg_dis"
  Demux/1 -> BusCreator/1  "PTC GearboxOut0 GearNoTrg"
  BusCreator/1 -> Out/1
  In/1 -> Demux/1

== system TorqueVect/CarMaker/IPG Vehicle/PowerTrain/PTControl Example/PTC GearBoxOut/CreateBus PTC GearboxOut1 ==
  In : Inport
  BusCreator : BusCreator  Inputs=12
  Demux : Demux  Outputs=12
      settings: DisplayOption=none
  Out : Outport  VectorParamsAs1DForOutWhenUnconnected=off
  wires:
  Demux/12 -> BusCreator/12  "PTC GearboxOut1 Clutch_dis Trq_out_trg"
  Demux/11 -> BusCreator/11  "PTC GearboxOut1 Clutch_dis rotv_out_trg"
  Demux/10 -> BusCreator/10  "PTC GearboxOut1 Clutch_dis Pos"
  Demux/9 -> BusCreator/9  "PTC GearboxOut1 Clutch Trq_out_trg"
  Demux/8 -> BusCreator/8  "PTC GearboxOut1 Clutch rotv_out_trg"
  Demux/7 -> BusCreator/7  "PTC GearboxOut1 Clutch Pos"
  Demux/6 -> BusCreator/6  "PTC GearboxOut1 Trq_out_trg"
  Demux/5 -> BusCreator/5  "PTC GearboxOut1 rotv_in_trg"
  Demux/4 -> BusCreator/4  "PTC GearboxOut1 i_trg"
  Demux/3 -> BusCreator/3  "PTC GearboxOut1 set_ParkBrake"
  Demux/2 -> BusCreator/2  "PTC GearboxOut1 GearNoTrg_dis"
  Demux/1 -> BusCreator/1  "PTC GearboxOut1 GearNoTrg"
  BusCreator/1 -> Out/1
  In/1 -> Demux/1

== system TorqueVect/CarMaker/IPG Vehicle/PowerTrain/PTControl Example/PTC GearBoxOut/CreateBus PTC GearboxOut10 ==
  In : Inport
  BusCreator : BusCreator  Inputs=12
  Demux : Demux  Outputs=12
      settings: DisplayOption=none
  Out : Outport  VectorParamsAs1DForOutWhenUnconnected=off
  wires:
  Demux/12 -> BusCreator/12  "PTC GearboxOut10 Clutch_dis Trq_out_trg"
  Demux/11 -> BusCreator/11  "PTC GearboxOut10 Clutch_dis rotv_out_trg"
  Demux/10 -> BusCreator/10  "PTC GearboxOut10 Clutch_dis Pos"
  Demux/9 -> BusCreator/9  "PTC GearboxOut10 Clutch Trq_out_trg"
  Demux/8 -> BusCreator/8  "PTC GearboxOut10 Clutch rotv_out_trg"
  Demux/7 -> BusCreator/7  "PTC GearboxOut10 Clutch Pos"
  Demux/6 -> BusCreator/6  "PTC GearboxOut10 Trq_out_trg"
  Demux/5 -> BusCreator/5  "PTC GearboxOut10 rotv_in_trg"
  Demux/4 -> BusCreator/4  "PTC GearboxOut10 i_trg"
  Demux/3 -> BusCreator/3  "PTC GearboxOut10 set_ParkBrake"
  Demux/2 -> BusCreator/2  "PTC GearboxOut10 GearNoTrg_dis"
  Demux/1 -> BusCreator/1  "PTC GearboxOut10 GearNoTrg"
  BusCreator/1 -> Out/1
  In/1 -> Demux/1

== system TorqueVect/CarMaker/IPG Vehicle/PowerTrain/PTControl Example/PTC GearBoxOut/CreateBus PTC GearboxOut11 ==
  In : Inport
  BusCreator : BusCreator  Inputs=12
  Demux : Demux  Outputs=12
      settings: DisplayOption=none
  Out : Outport  VectorParamsAs1DForOutWhenUnconnected=off
  wires:
  Demux/12 -> BusCreator/12  "PTC GearboxOut11 Clutch_dis Trq_out_trg"
  Demux/11 -> BusCreator/11  "PTC GearboxOut11 Clutch_dis rotv_out_trg"
  Demux/10 -> BusCreator/10  "PTC GearboxOut11 Clutch_dis Pos"
  Demux/9 -> BusCreator/9  "PTC GearboxOut11 Clutch Trq_out_trg"
  Demux/8 -> BusCreator/8  "PTC GearboxOut11 Clutch rotv_out_trg"
  Demux/7 -> BusCreator/7  "PTC GearboxOut11 Clutch Pos"
  Demux/6 -> BusCreator/6  "PTC GearboxOut11 Trq_out_trg"
  Demux/5 -> BusCreator/5  "PTC GearboxOut11 rotv_in_trg"
  Demux/4 -> BusCreator/4  "PTC GearboxOut11 i_trg"
  Demux/3 -> BusCreator/3  "PTC GearboxOut11 set_ParkBrake"
  Demux/2 -> BusCreator/2  "PTC GearboxOut11 GearNoTrg_dis"
  Demux/1 -> BusCreator/1  "PTC GearboxOut11 GearNoTrg"
  BusCreator/1 -> Out/1
  In/1 -> Demux/1

== system TorqueVect/CarMaker/IPG Vehicle/PowerTrain/PTControl Example/PTC GearBoxOut/CreateBus PTC GearboxOut2 ==
  In : Inport
  BusCreator : BusCreator  Inputs=12
  Demux : Demux  Outputs=12
      settings: DisplayOption=none
  Out : Outport  VectorParamsAs1DForOutWhenUnconnected=off
  wires:
  Demux/12 -> BusCreator/12  "PTC GearboxOut2 Clutch_dis Trq_out_trg"
  Demux/11 -> BusCreator/11  "PTC GearboxOut2 Clutch_dis rotv_out_trg"
  Demux/10 -> BusCreator/10  "PTC GearboxOut2 Clutch_dis Pos"
  Demux/9 -> BusCreator/9  "PTC GearboxOut2 Clutch Trq_out_trg"
  Demux/8 -> BusCreator/8  "PTC GearboxOut2 Clutch rotv_out_trg"
  Demux/7 -> BusCreator/7  "PTC GearboxOut2 Clutch Pos"
  Demux/6 -> BusCreator/6  "PTC GearboxOut2 Trq_out_trg"
  Demux/5 -> BusCreator/5  "PTC GearboxOut2 rotv_in_trg"
  Demux/4 -> BusCreator/4  "PTC GearboxOut2 i_trg"
  Demux/3 -> BusCreator/3  "PTC GearboxOut2 set_ParkBrake"
  Demux/2 -> BusCreator/2  "PTC GearboxOut2 GearNoTrg_dis"
  Demux/1 -> BusCreator/1  "PTC GearboxOut2 GearNoTrg"
  BusCreator/1 -> Out/1
  In/1 -> Demux/1

== system TorqueVect/CarMaker/IPG Vehicle/PowerTrain/PTControl Example/PTC GearBoxOut/CreateBus PTC GearboxOut3 ==
  In : Inport
  BusCreator : BusCreator  Inputs=12
  Demux : Demux  Outputs=12
      settings: DisplayOption=none
  Out : Outport  VectorParamsAs1DForOutWhenUnconnected=off
  wires:
  Demux/12 -> BusCreator/12  "PTC GearboxOut3 Clutch_dis Trq_out_trg"
  Demux/11 -> BusCreator/11  "PTC GearboxOut3 Clutch_dis rotv_out_trg"
  Demux/10 -> BusCreator/10  "PTC GearboxOut3 Clutch_dis Pos"
  Demux/9 -> BusCreator/9  "PTC GearboxOut3 Clutch Trq_out_trg"
  Demux/8 -> BusCreator/8  "PTC GearboxOut3 Clutch rotv_out_trg"
  Demux/7 -> BusCreator/7  "PTC GearboxOut3 Clutch Pos"
  Demux/6 -> BusCreator/6  "PTC GearboxOut3 Trq_out_trg"
  Demux/5 -> BusCreator/5  "PTC GearboxOut3 rotv_in_trg"
  Demux/4 -> BusCreator/4  "PTC GearboxOut3 i_trg"
  Demux/3 -> BusCreator/3  "PTC GearboxOut3 set_ParkBrake"
  Demux/2 -> BusCreator/2  "PTC GearboxOut3 GearNoTrg_dis"
  Demux/1 -> BusCreator/1  "PTC GearboxOut3 GearNoTrg"
  BusCreator/1 -> Out/1
  In/1 -> Demux/1

== system TorqueVect/CarMaker/IPG Vehicle/PowerTrain/PTControl Example/PTC GearBoxOut/CreateBus PTC GearboxOut4 ==
  In : Inport
  BusCreator : BusCreator  Inputs=12
  Demux : Demux  Outputs=12
      settings: DisplayOption=none
  Out : Outport  VectorParamsAs1DForOutWhenUnconnected=off
  wires:
  Demux/12 -> BusCreator/12  "PTC GearboxOut4 Clutch_dis Trq_out_trg"
  Demux/11 -> BusCreator/11  "PTC GearboxOut4 Clutch_dis rotv_out_trg"
  Demux/10 -> BusCreator/10  "PTC GearboxOut4 Clutch_dis Pos"
  Demux/9 -> BusCreator/9  "PTC GearboxOut4 Clutch Trq_out_trg"
  Demux/8 -> BusCreator/8  "PTC GearboxOut4 Clutch rotv_out_trg"
  Demux/7 -> BusCreator/7  "PTC GearboxOut4 Clutch Pos"
  Demux/6 -> BusCreator/6  "PTC GearboxOut4 Trq_out_trg"
  Demux/5 -> BusCreator/5  "PTC GearboxOut4 rotv_in_trg"
  Demux/4 -> BusCreator/4  "PTC GearboxOut4 i_trg"
  Demux/3 -> BusCreator/3  "PTC GearboxOut4 set_ParkBrake"
  Demux/2 -> BusCreator/2  "PTC GearboxOut4 GearNoTrg_dis"
  Demux/1 -> BusCreator/1  "PTC GearboxOut4 GearNoTrg"
  BusCreator/1 -> Out/1
  In/1 -> Demux/1

== system TorqueVect/CarMaker/IPG Vehicle/PowerTrain/PTControl Example/PTC GearBoxOut/CreateBus PTC GearboxOut5 ==
  In : Inport
  BusCreator : BusCreator  Inputs=12
  Demux : Demux  Outputs=12
      settings: DisplayOption=none
  Out : Outport  VectorParamsAs1DForOutWhenUnconnected=off
  wires:
  Demux/12 -> BusCreator/12  "PTC GearboxOut5 Clutch_dis Trq_out_trg"
  Demux/11 -> BusCreator/11  "PTC GearboxOut5 Clutch_dis rotv_out_trg"
  Demux/10 -> BusCreator/10  "PTC GearboxOut5 Clutch_dis Pos"
  Demux/9 -> BusCreator/9  "PTC GearboxOut5 Clutch Trq_out_trg"
  Demux/8 -> BusCreator/8  "PTC GearboxOut5 Clutch rotv_out_trg"
  Demux/7 -> BusCreator/7  "PTC GearboxOut5 Clutch Pos"
  Demux/6 -> BusCreator/6  "PTC GearboxOut5 Trq_out_trg"
  Demux/5 -> BusCreator/5  "PTC GearboxOut5 rotv_in_trg"
  Demux/4 -> BusCreator/4  "PTC GearboxOut5 i_trg"
  Demux/3 -> BusCreator/3  "PTC GearboxOut5 set_ParkBrake"
  Demux/2 -> BusCreator/2  "PTC GearboxOut5 GearNoTrg_dis"
  Demux/1 -> BusCreator/1  "PTC GearboxOut5 GearNoTrg"
  BusCreator/1 -> Out/1
  In/1 -> Demux/1

== system TorqueVect/CarMaker/IPG Vehicle/PowerTrain/PTControl Example/PTC GearBoxOut/CreateBus PTC GearboxOut6 ==
  In : Inport
  BusCreator : BusCreator  Inputs=12
  Demux : Demux  Outputs=12
      settings: DisplayOption=none
  Out : Outport  VectorParamsAs1DForOutWhenUnconnected=off
  wires:
  Demux/12 -> BusCreator/12  "PTC GearboxOut6 Clutch_dis Trq_out_trg"
  Demux/11 -> BusCreator/11  "PTC GearboxOut6 Clutch_dis rotv_out_trg"
  Demux/10 -> BusCreator/10  "PTC GearboxOut6 Clutch_dis Pos"
  Demux/9 -> BusCreator/9  "PTC GearboxOut6 Clutch Trq_out_trg"
  Demux/8 -> BusCreator/8  "PTC GearboxOut6 Clutch rotv_out_trg"
  Demux/7 -> BusCreator/7  "PTC GearboxOut6 Clutch Pos"
  Demux/6 -> BusCreator/6  "PTC GearboxOut6 Trq_out_trg"
  Demux/5 -> BusCreator/5  "PTC GearboxOut6 rotv_in_trg"
  Demux/4 -> BusCreator/4  "PTC GearboxOut6 i_trg"
  Demux/3 -> BusCreator/3  "PTC GearboxOut6 set_ParkBrake"
  Demux/2 -> BusCreator/2  "PTC GearboxOut6 GearNoTrg_dis"
  Demux/1 -> BusCreator/1  "PTC GearboxOut6 GearNoTrg"
  BusCreator/1 -> Out/1
  In/1 -> Demux/1

== system TorqueVect/CarMaker/IPG Vehicle/PowerTrain/PTControl Example/PTC GearBoxOut/CreateBus PTC GearboxOut7 ==
  In : Inport
  BusCreator : BusCreator  Inputs=12
  Demux : Demux  Outputs=12
      settings: DisplayOption=none
  Out : Outport  VectorParamsAs1DForOutWhenUnconnected=off
  wires:
  Demux/12 -> BusCreator/12  "PTC GearboxOut7 Clutch_dis Trq_out_trg"
  Demux/11 -> BusCreator/11  "PTC GearboxOut7 Clutch_dis rotv_out_trg"
  Demux/10 -> BusCreator/10  "PTC GearboxOut7 Clutch_dis Pos"
  Demux/9 -> BusCreator/9  "PTC GearboxOut7 Clutch Trq_out_trg"
  Demux/8 -> BusCreator/8  "PTC GearboxOut7 Clutch rotv_out_trg"
  Demux/7 -> BusCreator/7  "PTC GearboxOut7 Clutch Pos"
  Demux/6 -> BusCreator/6  "PTC GearboxOut7 Trq_out_trg"
  Demux/5 -> BusCreator/5  "PTC GearboxOut7 rotv_in_trg"
  Demux/4 -> BusCreator/4  "PTC GearboxOut7 i_trg"
  Demux/3 -> BusCreator/3  "PTC GearboxOut7 set_ParkBrake"
  Demux/2 -> BusCreator/2  "PTC GearboxOut7 GearNoTrg_dis"
  Demux/1 -> BusCreator/1  "PTC GearboxOut7 GearNoTrg"
  BusCreator/1 -> Out/1
  In/1 -> Demux/1

== system TorqueVect/CarMaker/IPG Vehicle/PowerTrain/PTControl Example/PTC GearBoxOut/CreateBus PTC GearboxOut8 ==
  In : Inport
  BusCreator : BusCreator  Inputs=12
  Demux : Demux  Outputs=12
      settings: DisplayOption=none
  Out : Outport  VectorParamsAs1DForOutWhenUnconnected=off
  wires:
  Demux/12 -> BusCreator/12  "PTC GearboxOut8 Clutch_dis Trq_out_trg"
  Demux/11 -> BusCreator/11  "PTC GearboxOut8 Clutch_dis rotv_out_trg"
  Demux/10 -> BusCreator/10  "PTC GearboxOut8 Clutch_dis Pos"
  Demux/9 -> BusCreator/9  "PTC GearboxOut8 Clutch Trq_out_trg"
  Demux/8 -> BusCreator/8  "PTC GearboxOut8 Clutch rotv_out_trg"
  Demux/7 -> BusCreator/7  "PTC GearboxOut8 Clutch Pos"
  Demux/6 -> BusCreator/6  "PTC GearboxOut8 Trq_out_trg"
  Demux/5 -> BusCreator/5  "PTC GearboxOut8 rotv_in_trg"
  Demux/4 -> BusCreator/4  "PTC GearboxOut8 i_trg"
  Demux/3 -> BusCreator/3  "PTC GearboxOut8 set_ParkBrake"
  Demux/2 -> BusCreator/2  "PTC GearboxOut8 GearNoTrg_dis"
  Demux/1 -> BusCreator/1  "PTC GearboxOut8 GearNoTrg"
  BusCreator/1 -> Out/1
  In/1 -> Demux/1

== system TorqueVect/CarMaker/IPG Vehicle/PowerTrain/PTControl Example/PTC GearBoxOut/CreateBus PTC GearboxOut9 ==
  In : Inport
  BusCreator : BusCreator  Inputs=12
  Demux : Demux  Outputs=12
      settings: DisplayOption=none
  Out : Outport  VectorParamsAs1DForOutWhenUnconnected=off
  wires:
  Demux/12 -> BusCreator/12  "PTC GearboxOut9 Clutch_dis Trq_out_trg"
  Demux/11 -> BusCreator/11  "PTC GearboxOut9 Clutch_dis rotv_out_trg"
  Demux/10 -> BusCreator/10  "PTC GearboxOut9 Clutch_dis Pos"
  Demux/9 -> BusCreator/9  "PTC GearboxOut9 Clutch Trq_out_trg"
  Demux/8 -> BusCreator/8  "PTC GearboxOut9 Clutch rotv_out_trg"
  Demux/7 -> BusCreator/7  "PTC GearboxOut9 Clutch Pos"
  Demux/6 -> BusCreator/6  "PTC GearboxOut9 Trq_out_trg"
  Demux/5 -> BusCreator/5  "PTC GearboxOut9 rotv_in_trg"
  Demux/4 -> BusCreator/4  "PTC GearboxOut9 i_trg"
  Demux/3 -> BusCreator/3  "PTC GearboxOut9 set_ParkBrake"
  Demux/2 -> BusCreator/2  "PTC GearboxOut9 GearNoTrg_dis"
  Demux/1 -> BusCreator/1  "PTC GearboxOut9 GearNoTrg"
  BusCreator/1 -> Out/1
  In/1 -> Demux/1

== system TorqueVect/CarMaker/IPG Vehicle/PowerTrain/PTControl Example/PTC MotorOut/CreateBus PTC MotorOut0 ==
  MotorOut0 : Inport
  BusCreator : BusCreator  Inputs=3
  Demux : Demux  Outputs=3
      settings: DisplayOption=none
  Out : Outport  VectorParamsAs1DForOutWhenUnconnected=off
  wires:
  Demux/3 -> BusCreator/3  "PTC MotorOut0 rotv_trg"
  Demux/2 -> BusCreator/2  "PTC MotorOut0 Trq_trg"
  Demux/1 -> BusCreator/1  "PTC MotorOut0 Load"
  BusCreator/1 -> Out/1
  MotorOut0/1 -> Demux/1

== system TorqueVect/CarMaker/IPG Vehicle/PowerTrain/PTControl Example/PTC MotorOut/CreateBus PTC MotorOut1 ==
  MotorOut1 : Inport
  BusCreator : BusCreator  Inputs=3
  Demux : Demux  Outputs=3
      settings: DisplayOption=none
  Out : Outport  VectorParamsAs1DForOutWhenUnconnected=off
  wires:
  Demux/3 -> BusCreator/3  "PTC MotorOut1 rotv_trg"
  Demux/2 -> BusCreator/2  "PTC MotorOut1 Trq_trg"
  Demux/1 -> BusCreator/1  "PTC MotorOut1 Load"
  BusCreator/1 -> Out/1
  MotorOut1/1 -> Demux/1

== system TorqueVect/CarMaker/IPG Vehicle/PowerTrain/PTControl Example/PTC MotorOut/CreateBus PTC MotorOut10 ==
  In : Inport
  BusCreator : BusCreator  Inputs=3
  Demux : Demux  Outputs=3
      settings: DisplayOption=none
  Out : Outport  VectorParamsAs1DForOutWhenUnconnected=off
  wires:
  Demux/3 -> BusCreator/3  "PTC MotorOut10 rotv_trg"
  Demux/2 -> BusCreator/2  "PTC MotorOut10 Trq_trg"
  Demux/1 -> BusCreator/1  "PTC MotorOut10 Load"
  BusCreator/1 -> Out/1
  In/1 -> Demux/1

== system TorqueVect/CarMaker/IPG Vehicle/PowerTrain/PTControl Example/PTC MotorOut/CreateBus PTC MotorOut11 ==
  In : Inport
  BusCreator : BusCreator  Inputs=3
  Demux : Demux  Outputs=3
      settings: DisplayOption=none
  Out : Outport  VectorParamsAs1DForOutWhenUnconnected=off
  wires:
  Demux/3 -> BusCreator/3  "PTC MotorOut11 rotv_trg"
  Demux/2 -> BusCreator/2  "PTC MotorOut11 Trq_trg"
  Demux/1 -> BusCreator/1  "PTC MotorOut11 Load"
  BusCreator/1 -> Out/1
  In/1 -> Demux/1

== system TorqueVect/CarMaker/IPG Vehicle/PowerTrain/PTControl Example/PTC MotorOut/CreateBus PTC MotorOut2 ==
  MotorOut2 : Inport
  BusCreator : BusCreator  Inputs=3
  Demux : Demux  Outputs=3
      settings: DisplayOption=none
  Out : Outport  VectorParamsAs1DForOutWhenUnconnected=off
  wires:
  Demux/3 -> BusCreator/3  "PTC MotorOut2 rotv_trg"
  Demux/2 -> BusCreator/2  "PTC MotorOut2 Trq_trg"
  Demux/1 -> BusCreator/1  "PTC MotorOut2 Load"
  BusCreator/1 -> Out/1
  MotorOut2/1 -> Demux/1

== system TorqueVect/CarMaker/IPG Vehicle/PowerTrain/PTControl Example/PTC MotorOut/CreateBus PTC MotorOut3 ==
  MotorOut3 : Inport
  BusCreator : BusCreator  Inputs=3
  Demux : Demux  Outputs=3
      settings: DisplayOption=none
  Out : Outport  VectorParamsAs1DForOutWhenUnconnected=off
  wires:
  Demux/3 -> BusCreator/3  "PTC MotorOut3 rotv_trg"
  Demux/2 -> BusCreator/2  "PTC MotorOut3 Trq_trg"
  Demux/1 -> BusCreator/1  "PTC MotorOut3 Load"
  BusCreator/1 -> Out/1
  MotorOut3/1 -> Demux/1

== system TorqueVect/CarMaker/IPG Vehicle/PowerTrain/PTControl Example/PTC MotorOut/CreateBus PTC MotorOut4 ==
  In : Inport
  BusCreator : BusCreator  Inputs=3
  Demux : Demux  Outputs=3
      settings: DisplayOption=none
  Out : Outport  VectorParamsAs1DForOutWhenUnconnected=off
  wires:
  Demux/3 -> BusCreator/3  "PTC MotorOut4 rotv_trg"
  Demux/2 -> BusCreator/2  "PTC MotorOut4 Trq_trg"
  Demux/1 -> BusCreator/1  "PTC MotorOut4 Load"
  BusCreator/1 -> Out/1
  In/1 -> Demux/1

== system TorqueVect/CarMaker/IPG Vehicle/PowerTrain/PTControl Example/PTC MotorOut/CreateBus PTC MotorOut5 ==
  In : Inport
  BusCreator : BusCreator  Inputs=3
  Demux : Demux  Outputs=3
      settings: DisplayOption=none
  Out : Outport  VectorParamsAs1DForOutWhenUnconnected=off
  wires:
  Demux/3 -> BusCreator/3  "PTC MotorOut5 rotv_trg"
  Demux/2 -> BusCreator/2  "PTC MotorOut5 Trq_trg"
  Demux/1 -> BusCreator/1  "PTC MotorOut5 Load"
  BusCreator/1 -> Out/1
  In/1 -> Demux/1

== system TorqueVect/CarMaker/IPG Vehicle/PowerTrain/PTControl Example/PTC MotorOut/CreateBus PTC MotorOut6 ==
  In : Inport
  BusCreator : BusCreator  Inputs=3
  Demux : Demux  Outputs=3
      settings: DisplayOption=none
  Out : Outport  VectorParamsAs1DForOutWhenUnconnected=off
  wires:
  Demux/3 -> BusCreator/3  "PTC MotorOut6 rotv_trg"
  Demux/2 -> BusCreator/2  "PTC MotorOut6 Trq_trg"
  Demux/1 -> BusCreator/1  "PTC MotorOut6 Load"
  BusCreator/1 -> Out/1
  In/1 -> Demux/1

== system TorqueVect/CarMaker/IPG Vehicle/PowerTrain/PTControl Example/PTC MotorOut/CreateBus PTC MotorOut7 ==
  In : Inport
  BusCreator : BusCreator  Inputs=3
  Demux : Demux  Outputs=3
      settings: DisplayOption=none
  Out : Outport  VectorParamsAs1DForOutWhenUnconnected=off
  wires:
  Demux/3 -> BusCreator/3  "PTC MotorOut7 rotv_trg"
  Demux/2 -> BusCreator/2  "PTC MotorOut7 Trq_trg"
  Demux/1 -> BusCreator/1  "PTC MotorOut7 Load"
  BusCreator/1 -> Out/1
  In/1 -> Demux/1
